simulink model "AltitudeHold"  (R2022b)
settings: Solver=VariableStepAuto  StartTime=0.0  StopTime=100  RelTol=1e-3
values from neighbouring files (symbols this model uses):
  Kq = k(2)    [Boeing747.m]
  Ktheta = k(3)    [Boeing747.m]
  Kw = k(1)    [Boeing747.m]
  TF_h = tf(U0*num_theta-num_w, conv([1 0], den_theta))    [Boeing747.m]
  U0 = 870.767717    [Boeing747.m]    (also in Gen_dimensional_derivatives.m = stb_coef(11))
undefined symbols (not defined in the file or in its folder): den_q, den_w, num_q, num_w
settings Model: Creator=^-^  LastModifiedBy=^-^

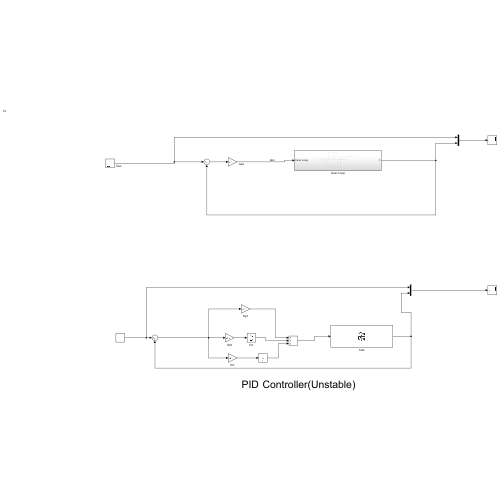
[thumbnail: Simulink's stored preview of the top-level diagram]
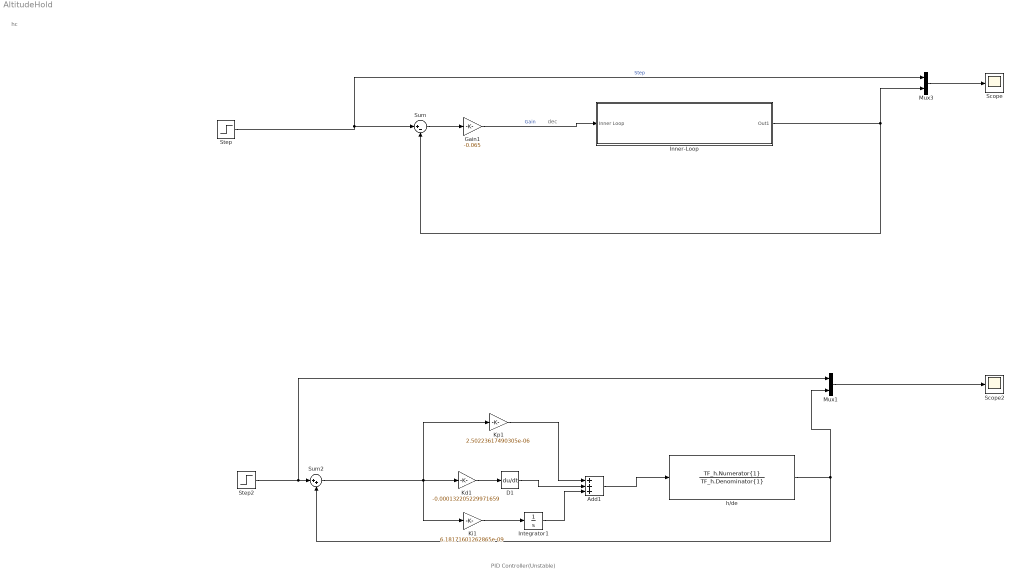
== system AltitudeHold ==
  note: hc
  note: dec
  note: PID Controller(Unstable)
  Add1 : Sum  Inputs=+++
  D1 : Derivative
  Gain1 : Gain  Gain=-0.065
  Inner-Loop : Subsystem
  Integrator1 : Integrator
  Kd1 : Gain  Gain=-0.000132205229971659
  Ki1 : Gain  Gain=6.18171601262865e-09
  Kp1 : Gain  Gain=2.50223617490305e-06
  Mux1 : Mux  Inputs=2
  Mux3 : Mux  Inputs=2
  Scope : Scope
  Scope2 : Scope
  Step : Step  SampleTime=0
  Step2 : Step  SampleTime=0
  Sum : Sum  Inputs=|+-
  Sum2 : Sum  Inputs=|++
  h/de : TransferFcn  Numerator=TF_h.Numerator{1}  Denominator=TF_h.Denominator{1}
  wires:
  Step/1 -> Mux3/1, Sum/1  "Step"
  Gain1/1 -> Inner-Loop/1(Inner Loop)  "Gain"
  Sum/1 -> Gain1/1
  Mux3/1 -> Scope/1
  Inner-Loop/1(Out1) -> Mux3/2, Sum/2
  Ki1/1 -> Integrator1/1
  Kp1/1 -> Add1/1
  Add1/1 -> h/de/1
  Kd1/1 -> D1/1
  h/de/1 -> Mux1/2, Sum2/2
  D1/1 -> Add1/2
  Mux1/1 -> Scope2/1
  Integrator1/1 -> Add1/3
  Sum2/1 -> Ki1/1, Kd1/1, Kp1/1
  Step2/1 -> Mux1/1, Sum2/1

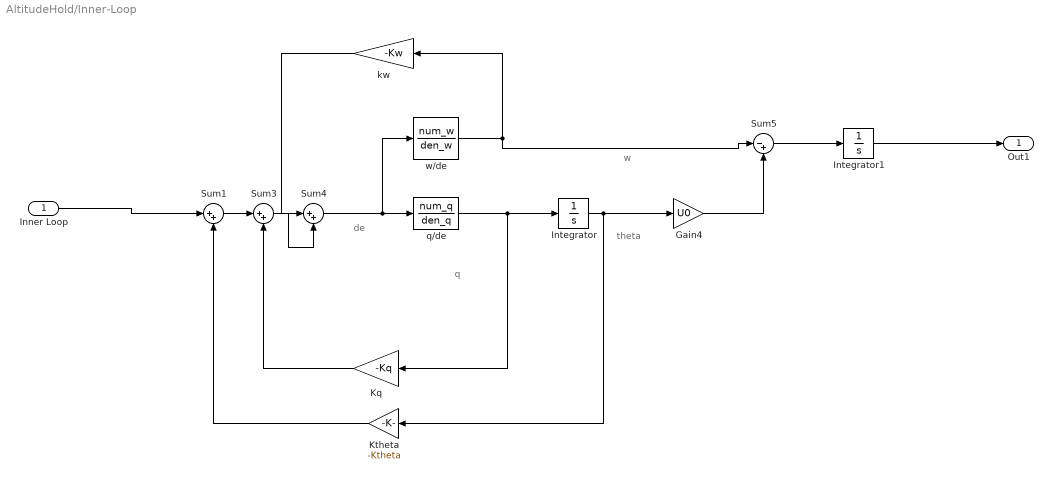
== system AltitudeHold/Inner-Loop ==
  note: de
  note: q
  note: w
  note: theta
  Inner Loop : Inport
  Gain4 : Gain  Gain=U0
  Integrator : Integrator
  Integrator1 : Integrator
  Kq : Gain  Gain=-Kq
  Ktheta : Gain  Gain=-Ktheta
  Sum1 : Sum  Inputs=|++
  Sum3 : Sum  Inputs=|++
  Sum4 : Sum  Inputs=|++
  Sum5 : Sum  Inputs=|-+
  kw : Gain  Gain=-Kw
  q/de : TransferFcn  Numerator=num_q  Denominator=den_q
  w/de : TransferFcn  Numerator=num_w  Denominator=den_w
  Out1 : Outport
  wires:
  q/de/1 -> Kq/1, Integrator/1
  kw/1 -> Sum4/1
  w/de/1 -> Sum5/1, kw/1
  Inner Loop/1 -> Sum1/1
  Ktheta/1 -> Sum1/2
  Sum5/1 -> Integrator1/1
  Integrator/1 -> Ktheta/1, Gain4/1
  Sum4/1 -> q/de/1, w/de/1
  Gain4/1 -> Sum5/2
  Sum1/1 -> Sum3/1
  Sum3/1 -> Sum4/2
  Kq/1 -> Sum3/2
  Integrator1/1 -> Out1/1
